simulink model "ThdRwRtStCshnFldIsPosChk"  (R2018b)
settings: Solver=FixedStepDiscrete  StartTime=0.0  StopTime=10.0  FixedStep=0.01  RelTol=1e-3
undefined symbols (not defined in the file or in its folder): KeSMSuThrdRwCushFoldPosDelta_Val, KeSMSuThrdRwCushFoldPosTolr_Val, KeSMSuVehicleModelConfig_Val
libraries: StIsPosChkLib x8, simulink x5
settings Model: Creator=sn2xws  LastModifiedBy=sn55gm
settings Model: ModifiedHistory=|
  | 2024.3.14
  | V2.3.0
  | Bug 813950 童锁Lock，Mode1_Easy Entry Mode 不应调用失败
  | 2024.6.25
  | V3.0.0 557模式流程V1.6
  | 2024.9.6 V3.0.1 新增Md56
  | 2025.2.19 V3.8.0 Bug 991386 Md1 三排占座时未移动且报了成功
  | 25.7.1 v3.13.0 新增Md61 Md62
settings DataIOCC: SaveFormat=StructureWithTime
settings OptimizationCC: DefaultParameterBehavior=Inlined  EnhancedBackFolding=on  PassReuseOutputArgsAs=Individual arguments  ZeroExternalMemoryAtStartup=off  ZeroInternalMemoryAtStartup=off  OptimizeBlockOrder=speed  DifferentSizesBufferReuse=on  OptimizationCustomize=off
settings DebuggingCC: ParameterTunabilityLossMsg=error
settings ModelReferenceCC: ModelReferenceNumInstancesAllowed=Single
settings SFSimCC: MATLABDynamicMemAlloc=off
settings RTWCC: SystemTargetFile=autosar.tlc  GenCodeOnly=on  TemplateMakefile=ert_default_tmf  Description=AUTOSAR  GenerateReport=on  IncludeHyperlinkInReport=on  LaunchReport=on  GenerateTraceInfo=on  GenerateTraceReport=on  GenerateTraceReportSl=on  GenerateTraceReportSf=on  GenerateTraceReportEml=on
settings CodeAppCC: ForceParamTrailComments=on  IgnoreCustomStorageClasses=off  OperatorAnnotations=on  SimulinkDataObjDesc=on  SFDataObjDesc=on  InsertBlockDesc=on
settings STFCustomTargetCC: TargetLangStandard=C99 (ISO)  MultiwordLength=256  ParMdlRefBuildCompliant=on  CompOptLevelCompliant=on  IncludeMdlTerminateFcn=off  CombineOutputUpdateFcns=on  SuppressErrorStatus=on  ERTCustomFileBanners=on  SupportNonFinite=off  SupportComplex=off  SupportContinuousTime=off  SupportNonInlinedSFcns=off  RemoveResetFunc=on  MATLABClassNameForMDSCustomization=Simulink.SoftwareTarget.ERTCustomization  AutosarCompliant=on  UseToolchainInfoCompliant=on  LookupTableObjectStructAxisOrder=2,1,3,4,...  LUTObjectStructOrderEvenSpacing=Size,Table,Breakpoints  SystemTargetFile=autosar.tlc
settings ERTTargetCC: TargetLangStandard=C99 (ISO)  ConcurrentExecutionCompliant=off  IncludeMdlTerminateFcn=off  SuppressErrorStatus=on  SupportNonFinite=off  SupportComplex=off  ModelStepFunctionPrototypeControlCompliant=off  CPPClassGenCompliant=off  AutosarCompliant=on  LookupTableObjectStructAxisOrder=2,1,3,4,...  LUTObjectStructOrderEvenSpacing=Size,Table,Breakpoints  InlinedParameterPlacement=NonHierarchical  ERTCustomFileTemplate=example_file_process.tlc  ERTFilePackagingFormat=Compact

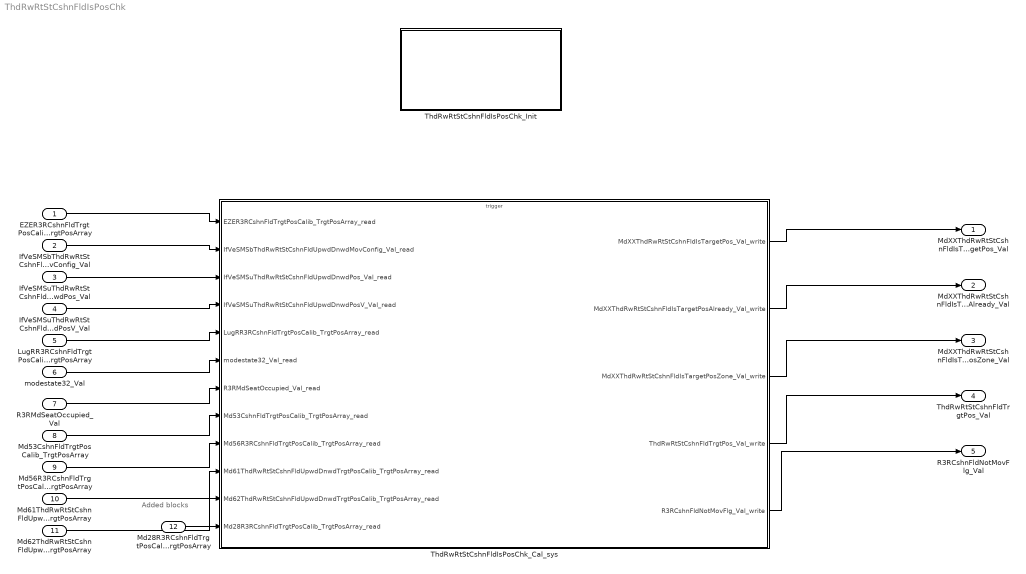
== system ThdRwRtStCshnFldIsPosChk ==
  note: Added blocks
  EZER3RCshnFldTrgtPosCalib_TrgtPosArray : Inport  Description=|  OutDataTypeStr=uint16  PortDimensions=3
      | 0:Pos
      | 1:Max
      | 2:Min
  IfVeSMSbThdRwRtStCshnFldUpwdDnwdMovConfig_Val : Inport  Port=2  OutDataTypeStr=boolean  PortDimensions=1
  IfVeSMSuThdRwRtStCshnFldUpwdDnwdPos_Val : Inport  Port=3  OutDataTypeStr=uint16  PortDimensions=1
  IfVeSMSuThdRwRtStCshnFldUpwdDnwdPosV_Val : Inport  Port=4  OutDataTypeStr=boolean  PortDimensions=1
  LugRR3RCshnFldTrgtPosCalib_TrgtPosArray : Inport  Description=|  Port=5  OutDataTypeStr=uint16  PortDimensions=3
      | 0:Pos
      | 1:Max
      | 2:Min
  modestate32_Val : Inport  Port=6  OutDataTypeStr=uint32  PortDimensions=1
  R3RMdSeatOccupied_Val : Inport  Port=7  OutDataTypeStr=boolean  PortDimensions=1
  Md53CshnFldTrgtPosCalib_TrgtPosArray : Inport  Description=|  Port=8  OutDataTypeStr=uint16  PortDimensions=3
      | 0:Pos
      | 1:Max
      | 2:Min
  Md56R3RCshnFldTrgtPosCalib_TrgtPosArray : Inport  Description=|  Port=9  OutDataTypeStr=uint16  PortDimensions=3
      | 0:Pos
      | 1:Max
      | 2:Min
  Md61ThdRwRtStCshnFldUpwdDnwdTrgtPosCalib_TrgtPosArray : Inport  Description=|  Port=10  OutDataTypeStr=uint16  PortDimensions=3
      | 0:Pos
      | 1:Max
      | 2:Min
  Md62ThdRwRtStCshnFldUpwdDnwdTrgtPosCalib_TrgtPosArray : Inport  Description=|  Port=11  OutDataTypeStr=uint16  PortDimensions=3
      | 0:Pos
      | 1:Max
      | 2:Min
  Md28R3RCshnFldTrgtPosCalib_TrgtPosArray : Inport  Description=|  Port=12  OutDataTypeStr=uint16  PortDimensions=3
      | 0:Pos
      | 1:Max
      | 2:Min
  ThdRwRtStCshnFldIsPosChk_Cal_sys : Subsystem
  ThdRwRtStCshnFldIsPosChk_Init : Subsystem
  MdXXThdRwRtStCshnFldIsTargetPos_Val : Outport  OutDataTypeStr=uint32  PortDimensions=1
  MdXXThdRwRtStCshnFldIsTargetPosAlready_Val : Outport  Port=2  OutDataTypeStr=uint32  PortDimensions=1
  MdXXThdRwRtStCshnFldIsTargetPosZone_Val : Outport  Port=3  OutDataTypeStr=uint32  PortDimensions=1
  ThdRwRtStCshnFldTrgtPos_Val : Outport  Port=4  OutDataTypeStr=uint16  PortDimensions=1
  R3RCshnFldNotMovFlg_Val : Outport  Port=5  OutDataTypeStr=boolean  PortDimensions=1
  wires:
  EZER3RCshnFldTrgtPosCalib_TrgtPosArray/1 -> ThdRwRtStCshnFldIsPosChk_Cal_sys/1(EZER3RCshnFldTrgtPosCalib_TrgtPosArray_read)
  IfVeSMSbThdRwRtStCshnFldUpwdDnwdMovConfig_Val/1 -> ThdRwRtStCshnFldIsPosChk_Cal_sys/2(IfVeSMSbThdRwRtStCshnFldUpwdDnwdMovConfig_Val_read)
  IfVeSMSuThdRwRtStCshnFldUpwdDnwdPos_Val/1 -> ThdRwRtStCshnFldIsPosChk_Cal_sys/3(IfVeSMSuThdRwRtStCshnFldUpwdDnwdPos_Val_read)
  IfVeSMSuThdRwRtStCshnFldUpwdDnwdPosV_Val/1 -> ThdRwRtStCshnFldIsPosChk_Cal_sys/4(IfVeSMSuThdRwRtStCshnFldUpwdDnwdPosV_Val_read)
  LugRR3RCshnFldTrgtPosCalib_TrgtPosArray/1 -> ThdRwRtStCshnFldIsPosChk_Cal_sys/5(LugRR3RCshnFldTrgtPosCalib_TrgtPosArray_read)
  modestate32_Val/1 -> ThdRwRtStCshnFldIsPosChk_Cal_sys/6(modestate32_Val_read)
  ThdRwRtStCshnFldIsPosChk_Cal_sys/1(MdXXThdRwRtStCshnFldIsTargetPos_Val_write) -> MdXXThdRwRtStCshnFldIsTargetPos_Val/1
  ThdRwRtStCshnFldIsPosChk_Cal_sys/2(MdXXThdRwRtStCshnFldIsTargetPosAlready_Val_write) -> MdXXThdRwRtStCshnFldIsTargetPosAlready_Val/1
  ThdRwRtStCshnFldIsPosChk_Cal_sys/3(MdXXThdRwRtStCshnFldIsTargetPosZone_Val_write) -> MdXXThdRwRtStCshnFldIsTargetPosZone_Val/1
  ThdRwRtStCshnFldIsPosChk_Cal_sys/4(ThdRwRtStCshnFldTrgtPos_Val_write) -> ThdRwRtStCshnFldTrgtPos_Val/1
  R3RMdSeatOccupied_Val/1 -> ThdRwRtStCshnFldIsPosChk_Cal_sys/7(R3RMdSeatOccupied_Val_read)
  Md53CshnFldTrgtPosCalib_TrgtPosArray/1 -> ThdRwRtStCshnFldIsPosChk_Cal_sys/8(Md53CshnFldTrgtPosCalib_TrgtPosArray_read)
  ThdRwRtStCshnFldIsPosChk_Cal_sys/5(R3RCshnFldNotMovFlg_Val_write) -> R3RCshnFldNotMovFlg_Val/1
  Md56R3RCshnFldTrgtPosCalib_TrgtPosArray/1 -> ThdRwRtStCshnFldIsPosChk_Cal_sys/9(Md56R3RCshnFldTrgtPosCalib_TrgtPosArray_read)
  Md61ThdRwRtStCshnFldUpwdDnwdTrgtPosCalib_TrgtPosArray/1 -> ThdRwRtStCshnFldIsPosChk_Cal_sys/10(Md61ThdRwRtStCshnFldUpwdDnwdTrgtPosCalib_TrgtPosArray_read)
  Md62ThdRwRtStCshnFldUpwdDnwdTrgtPosCalib_TrgtPosArray/1 -> ThdRwRtStCshnFldIsPosChk_Cal_sys/11(Md62ThdRwRtStCshnFldUpwdDnwdTrgtPosCalib_TrgtPosArray_read)
  Md28R3RCshnFldTrgtPosCalib_TrgtPosArray/1 -> ThdRwRtStCshnFldIsPosChk_Cal_sys/12(Md28R3RCshnFldTrgtPosCalib_TrgtPosArray_read)

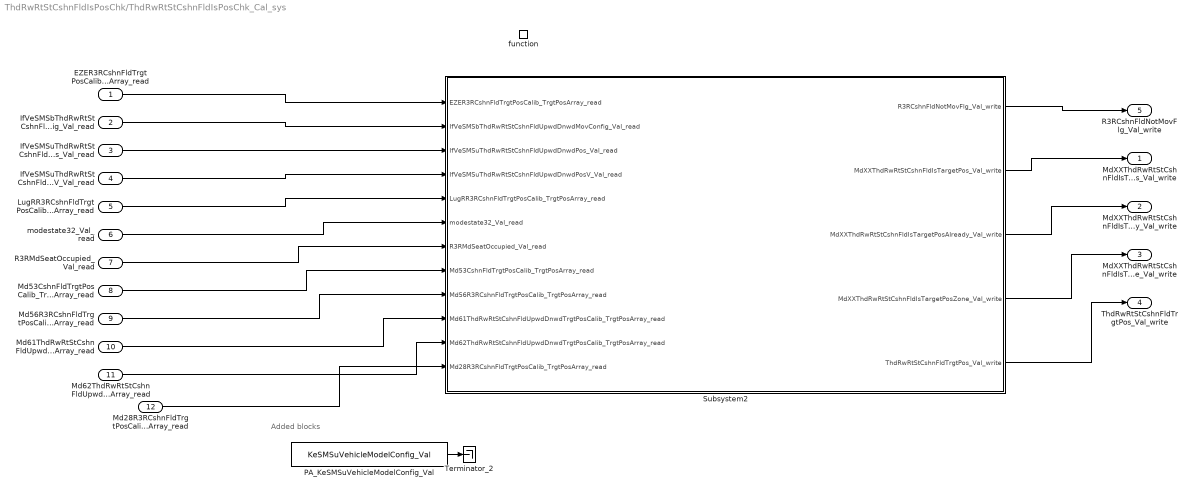
== system ThdRwRtStCshnFldIsPosChk/ThdRwRtStCshnFldIsPosChk_Cal_sys ==
  note: Added blocks
  EZER3RCshnFldTrgtPosCalib_TrgtPosArray_read : Inport
  IfVeSMSbThdRwRtStCshnFldUpwdDnwdMovConfig_Val_read : Inport  Port=2
  IfVeSMSuThdRwRtStCshnFldUpwdDnwdPos_Val_read : Inport  Port=3
  IfVeSMSuThdRwRtStCshnFldUpwdDnwdPosV_Val_read : Inport  Port=4
  LugRR3RCshnFldTrgtPosCalib_TrgtPosArray_read : Inport  Port=5
  modestate32_Val_read : Inport  Port=6
  R3RMdSeatOccupied_Val_read : Inport  Port=7
  Md53CshnFldTrgtPosCalib_TrgtPosArray_read : Inport  Port=8
  Md56R3RCshnFldTrgtPosCalib_TrgtPosArray_read : Inport  Port=9
  Md61ThdRwRtStCshnFldUpwdDnwdTrgtPosCalib_TrgtPosArray_read : Inport  Port=10
  Md62ThdRwRtStCshnFldUpwdDnwdTrgtPosCalib_TrgtPosArray_read : Inport  Port=11
  Md28R3RCshnFldTrgtPosCalib_TrgtPosArray_read : Inport  Port=12
  function : TriggerPort  TriggerType=function-call  IsSimulinkFunction=on  FunctionName=ThdRwRtStCshnFldIsPosChk_Cal  VariantControl=(inherit)
  PA_KeSMSuVehicleModelConfig_Val : Constant  Value=KeSMSuVehicleModelConfig_Val
  Subsystem2 : Subsystem
  Terminator_2 : Terminator
  MdXXThdRwRtStCshnFldIsTargetPos_Val_write : Outport
      settings: EnsureOutportIsVirtual=on
  MdXXThdRwRtStCshnFldIsTargetPosAlready_Val_write : Outport  Port=2
      settings: EnsureOutportIsVirtual=on
  MdXXThdRwRtStCshnFldIsTargetPosZone_Val_write : Outport  Port=3
      settings: EnsureOutportIsVirtual=on
  ThdRwRtStCshnFldTrgtPos_Val_write : Outport  Port=4
      settings: EnsureOutportIsVirtual=on
  R3RCshnFldNotMovFlg_Val_write : Outport  Port=5
      settings: EnsureOutportIsVirtual=on
  wires:
  Subsystem2/5(ThdRwRtStCshnFldTrgtPos_Val_write) -> ThdRwRtStCshnFldTrgtPos_Val_write/1
  Subsystem2/2(MdXXThdRwRtStCshnFldIsTargetPos_Val_write) -> MdXXThdRwRtStCshnFldIsTargetPos_Val_write/1
  Subsystem2/3(MdXXThdRwRtStCshnFldIsTargetPosAlready_Val_write) -> MdXXThdRwRtStCshnFldIsTargetPosAlready_Val_write/1
  Subsystem2/4(MdXXThdRwRtStCshnFldIsTargetPosZone_Val_write) -> MdXXThdRwRtStCshnFldIsTargetPosZone_Val_write/1
  EZER3RCshnFldTrgtPosCalib_TrgtPosArray_read/1 -> Subsystem2/1(EZER3RCshnFldTrgtPosCalib_TrgtPosArray_read)
  IfVeSMSbThdRwRtStCshnFldUpwdDnwdMovConfig_Val_read/1 -> Subsystem2/2(IfVeSMSbThdRwRtStCshnFldUpwdDnwdMovConfig_Val_read)
  IfVeSMSuThdRwRtStCshnFldUpwdDnwdPos_Val_read/1 -> Subsystem2/3(IfVeSMSuThdRwRtStCshnFldUpwdDnwdPos_Val_read)
  IfVeSMSuThdRwRtStCshnFldUpwdDnwdPosV_Val_read/1 -> Subsystem2/4(IfVeSMSuThdRwRtStCshnFldUpwdDnwdPosV_Val_read)
  LugRR3RCshnFldTrgtPosCalib_TrgtPosArray_read/1 -> Subsystem2/5(LugRR3RCshnFldTrgtPosCalib_TrgtPosArray_read)
  modestate32_Val_read/1 -> Subsystem2/6(modestate32_Val_read)
  R3RMdSeatOccupied_Val_read/1 -> Subsystem2/7(R3RMdSeatOccupied_Val_read)
  Md53CshnFldTrgtPosCalib_TrgtPosArray_read/1 -> Subsystem2/8(Md53CshnFldTrgtPosCalib_TrgtPosArray_read)
  Subsystem2/1(R3RCshnFldNotMovFlg_Val_write) -> R3RCshnFldNotMovFlg_Val_write/1
  Md56R3RCshnFldTrgtPosCalib_TrgtPosArray_read/1 -> Subsystem2/9(Md56R3RCshnFldTrgtPosCalib_TrgtPosArray_read)
  Md61ThdRwRtStCshnFldUpwdDnwdTrgtPosCalib_TrgtPosArray_read/1 -> Subsystem2/10(Md61ThdRwRtStCshnFldUpwdDnwdTrgtPosCalib_TrgtPosArray_read)
  Md62ThdRwRtStCshnFldUpwdDnwdTrgtPosCalib_TrgtPosArray_read/1 -> Subsystem2/11(Md62ThdRwRtStCshnFldUpwdDnwdTrgtPosCalib_TrgtPosArray_read)
  Md28R3RCshnFldTrgtPosCalib_TrgtPosArray_read/1 -> Subsystem2/12(Md28R3RCshnFldTrgtPosCalib_TrgtPosArray_read)
  PA_KeSMSuVehicleModelConfig_Val/1 -> Terminator_2/1

== system ThdRwRtStCshnFldIsPosChk/ThdRwRtStCshnFldIsPosChk_Init ==
  note: Added blocks
  note: Added blocks
  note: Added blocks
  Event Listener : EventListener  EventName=reset
  PA_KeSMSuThrdRwCushFoldPosDelta_Val : Constant  Value=KeSMSuThrdRwCushFoldPosDelta_Val
  PA_KeSMSuThrdRwCushFoldPosTolr_Val : Constant  Value=KeSMSuThrdRwCushFoldPosTolr_Val
  PA_KeSMSuVehicleModelConfig_Val : Constant  Value=KeSMSuVehicleModelConfig_Val
  Terminator_1 : Terminator
  Terminator_2 : Terminator
  Terminator_3 : Terminator
  wires:
  PA_KeSMSuThrdRwCushFoldPosDelta_Val/1 -> Terminator_1/1
  PA_KeSMSuThrdRwCushFoldPosTolr_Val/1 -> Terminator_2/1
  PA_KeSMSuVehicleModelConfig_Val/1 -> Terminator_3/1

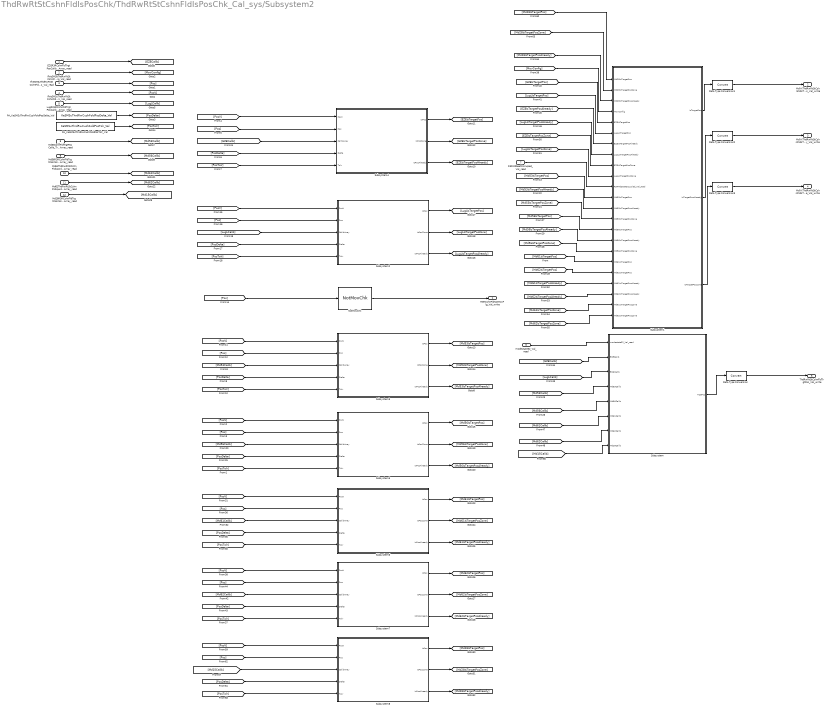
== system ThdRwRtStCshnFldIsPosChk/ThdRwRtStCshnFldIsPosChk_Cal_sys/Subsystem2 ==
  EZER3RCshnFldTrgtPosCalib_TrgtPosArray_read : Inport
  IfVeSMSbThdRwRtStCshnFldUpwdDnwdMovConfig_Val_read : Inport  Port=2
  IfVeSMSuThdRwRtStCshnFldUpwdDnwdPos_Val_read : Inport  Port=3
  IfVeSMSuThdRwRtStCshnFldUpwdDnwdPosV_Val_read : Inport  Port=4
  LugRR3RCshnFldTrgtPosCalib_TrgtPosArray_read : Inport  Port=5
  modestate32_Val_read : Inport  Port=6
  R3RMdSeatOccupied_Val_read : Inport  Port=7
  Md53CshnFldTrgtPosCalib_TrgtPosArray_read : Inport  Port=8
  Md56R3RCshnFldTrgtPosCalib_TrgtPosArray_read : Inport  Port=9
  Md61ThdRwRtStCshnFldUpwdDnwdTrgtPosCalib_TrgtPosArray_read : Inport  Port=10
  Md62ThdRwRtStCshnFldUpwdDnwdTrgtPosCalib_TrgtPosArray_read : Inport  Port=11
  Md28R3RCshnFldTrgtPosCalib_TrgtPosArray_read : Inport  Port=12
  Data Type Conversion{,1..3} (4 alike) : DataTypeConversion
  NotMovChk : StIsPosChkLib/NotMovChk  SystemSampleTime=-1
  PA_KeSMSuThrdRwCushFoldPosDelta_Val : Constant  Value=KeSMSuThrdRwCushFoldPosDelta_Val
  PA_KeSMSuThrdRwCushFoldPosTolr_Val : Constant  Value=KeSMSuThrdRwCushFoldPosTolr_Val
  Subsystem : Subsystem
  Subsystem1 : Subsystem
  Subsystem2 : Subsystem
  Subsystem3 : Subsystem
  Subsystem4 : Subsystem
  Subsystem5 : Subsystem
  Subsystem6 : Subsystem
  Subsystem7 : Subsystem
  Subsystem8 : Subsystem
  R3RCshnFldNotMovFlg_Val_write : Outport
      settings: EnsureOutportIsVirtual=on
  MdXXThdRwRtStCshnFldIsTargetPos_Val_write : Outport  Port=2
      settings: EnsureOutportIsVirtual=on
  MdXXThdRwRtStCshnFldIsTargetPosAlready_Val_write : Outport  Port=3
      settings: EnsureOutportIsVirtual=on
  MdXXThdRwRtStCshnFldIsTargetPosZone_Val_write : Outport  Port=4
      settings: EnsureOutportIsVirtual=on
  ThdRwRtStCshnFldTrgtPos_Val_write : Outport  Port=5
      settings: EnsureOutportIsVirtual=on
  wires:
  [LugLCalib] -> Subsystem/3(EZQCalib)
  Subsystem1/3(IsTargetPosZone) -> Data Type Conversion3/1
  [EZEIsTargetPosZone] -> Subsystem1/9(EZEIsTargetPosZone)
  [EZECalib] -> Subsystem/2(EZECalib)
  NotMovChk/1 -> R3RCshnFldNotMovFlg_Val_write/1
  [EZEIsTargetPosAlready] -> Subsystem1/7(EZEIsTargetPosAlready)
  [LugLIsTargetPosAlready] -> Subsystem1/8(LugLIsTargetPosAlready)
  Subsystem2/2(IsPosZone) -> [LugLIsTargetPosZone]
  modestate32_Val_read/1 -> Subsystem/1(modestate32_Val_read)
  Data Type Conversion1/1 -> MdXXThdRwRtStCshnFldIsTargetPos_Val_write/1
  Subsystem2/1(IsPos) -> [LugLIsTargetPos]
  Subsystem/1(TrgtPos) -> Data Type Conversion/1
  Subsystem4/3(IsPosAlready) -> [EZEIsTargetPosAlready]
  [EZECalib] -> Subsystem4/3(CalibArray)
  [LugLIsTargetPos] -> Subsystem1/6(LugLIsTargetPos)
  [EZEIsTargetPos] -> Subsystem1/5(EZEIsTargetPos)
  Subsystem1/1(IsTargetPos) -> Data Type Conversion1/1
  Subsystem4/1(IsPos) -> [EZEIsTargetPos]
  Data Type Conversion2/1 -> MdXXThdRwRtStCshnFldIsTargetPosAlready_Val_write/1
  [PosV] -> Subsystem4/1(PosV)
  [LugLCalib] -> Subsystem2/3(CalibArray)
  [LugLIsTargetPosZone] -> Subsystem1/10(LugLIsTargetPosZone)
  [PosDelta] -> Subsystem4/4(Delta)
  Data Type Conversion/1 -> ThdRwRtStCshnFldTrgtPos_Val_write/1
  PA_KeSMSuThrdRwCushFoldPosDelta_Val/1 -> [PosDelta]
  [PosDelta] -> Subsystem2/4(Delta)
  EZER3RCshnFldTrgtPosCalib_TrgtPosArray_read/1 -> [EZECalib]
  IfVeSMSbThdRwRtStCshnFldUpwdDnwdMovConfig_Val_read/1 -> [MovConfig]
  IfVeSMSuThdRwRtStCshnFldUpwdDnwdPosV_Val_read/1 -> [PosV]
  IfVeSMSuThdRwRtStCshnFldUpwdDnwdPos_Val_read/1 -> [Pos]
  [PosTolr] -> Subsystem4/5(Tolr)
  Subsystem2/3(IsPosAlready) -> [LugLIsTargetPosAlready]
  LugRR3RCshnFldTrgtPosCalib_TrgtPosArray_read/1 -> [LugLCalib]
  [Pos] -> Subsystem2/2(Pos)
  PA_KeSMSuThrdRwCushFoldPosTolr_Val/1 -> [PosTolr]
  Subsystem4/2(IsPosZone) -> [EZEIsTargetPosZone]
  [PosV] -> Subsystem2/1(PosV)
  Subsystem1/2(IsTargetPosAlready) -> Data Type Conversion2/1
  [PosTolr] -> Subsystem2/5(Tolr)
  [MovConfig] -> Subsystem1/4(MovConfig)
  [Pos] -> NotMovChk/1
  [Pos] -> Subsystem4/2(Pos)
  Data Type Conversion3/1 -> MdXXThdRwRtStCshnFldIsTargetPosZone_Val_write/1
  R3RMdSeatOccupied_Val_read/1 -> Subsystem1/11(R3RMdSeatOccupied_Val_read)
  Md53CshnFldTrgtPosCalib_TrgtPosArray_read/1 -> [Md53Calib]
  [Md53Calib] -> Subsystem3/3(CalibArray)
  [PosTolr] -> Subsystem3/5(Tolr)
  [PosDelta] -> Subsystem3/4(Delta)
  [PosV] -> Subsystem3/1(PosV)
  [Pos] -> Subsystem3/2(Pos)
  Subsystem3/3(IsPosAlready) -> [Md53IsTargetPosAlready]
  Subsystem3/1(IsPos) -> [Md53IsTargetPos]
  Subsystem3/2(IsPosZone) -> [Md53IsTargetPosZone]
  [Md53Calib] -> Subsystem/4(Md53Calib)
  [Md53IsTargetPos] -> Subsystem1/12(Md53IsTargetPos)
  [Md53IsTargetPosAlready] -> Subsystem1/13(Md53IsTargetPosAlready)
  [Md53IsTargetPosZone] -> Subsystem1/14(Md53IsTargetPosZone)
  Md56R3RCshnFldTrgtPosCalib_TrgtPosArray_read/1 -> [Md56Calib]
  Subsystem5/2(IsPosZone) -> [Md56IsTargetPosZone]
  Subsystem5/1(IsPos) -> [Md56IsTargetPos]
  Subsystem5/3(IsPosAlready) -> [Md56IsTargetPosAlready]
  [Pos] -> Subsystem5/2(Pos)
  [PosV] -> Subsystem5/1(PosV)
  [PosDelta] -> Subsystem5/4(Delta)
  [PosTolr] -> Subsystem5/5(Tolr)
  [Md56Calib] -> Subsystem5/3(CalibArray)
  [Md56Calib] -> Subsystem/5(Md56Calib)
  [Md56IsTargetPos] -> Subsystem1/15(Md56IsTargetPos)
  [Md56IsTargetPosAlready] -> Subsystem1/16(Md56IsTargetPosAlready)
  [Md56IsTargetPosZone] -> Subsystem1/17(Md56IsTargetPosZone)
  Md62ThdRwRtStCshnFldUpwdDnwdTrgtPosCalib_TrgtPosArray_read/1 -> [Md62Calib]
  Md61ThdRwRtStCshnFldUpwdDnwdTrgtPosCalib_TrgtPosArray_read/1 -> [Md61Calib]
  [Md61Calib] -> Subsystem6/3(CalibArray)
  [PosTolr] -> Subsystem6/5(Tolr)
  [PosDelta] -> Subsystem6/4(Delta)
  [PosV] -> Subsystem6/1(PosV)
  [Pos] -> Subsystem6/2(Pos)
  Subsystem6/3(IsPosAlready) -> [Md61IsTargetPosAlready]
  Subsystem6/1(IsPos) -> [Md61IsTargetPos]
  Subsystem6/2(IsPosZone) -> [Md61IsTargetPosZone]
  Subsystem7/2(IsPosZone) -> [Md62IsTargetPosZone]
  Subsystem7/1(IsPos) -> [Md62IsTargetPos]
  Subsystem7/3(IsPosAlready) -> [Md62IsTargetPosAlready]
  [Pos] -> Subsystem7/2(Pos)
  [PosV] -> Subsystem7/1(PosV)
  [PosDelta] -> Subsystem7/4(Delta)
  [PosTolr] -> Subsystem7/5(Tolr)
  [Md62Calib] -> Subsystem7/3(CalibArray)
  [Md62Calib] -> Subsystem/7(Md62Calib)
  [Md61Calib] -> Subsystem/6(Md61Calib)
  [Md61IsTargetPos] -> Subsystem1/18(Md61IsTargetPos)
  [Md62IsTargetPos] -> Subsystem1/19(Md62IsTargetPos)
  [Md61IsTargetPosAlready] -> Subsystem1/20(Md61IsTargetPosAlready)
  [Md62IsTargetPosAlready] -> Subsystem1/21(Md62IsTargetPosAlready)
  [Md61IsTargetPosZone] -> Subsystem1/22(Md61IsTargetPosZone)
  [Md62IsTargetPosZone] -> Subsystem1/23(Md62IsTargetPosZone)
  Md28R3RCshnFldTrgtPosCalib_TrgtPosArray_read/1 -> [Md15Calib]
  [PosTolr] -> Subsystem8/5(Tolr)
  Subsystem8/3(IsPosAlready) -> [Md28IsTargetPosAlready]
  [PosV] -> Subsystem8/1(PosV)
  [Pos] -> Subsystem8/2(Pos)
  [PosDelta] -> Subsystem8/4(Delta)
  [Md15Calib] -> Subsystem8/3(CalibArray)
  Subsystem8/1(IsPos) -> [Md28IsTargetPos]
  Subsystem8/2(IsPosZone) -> [Md28IsTargetPosZone]
  [Md28IsTargetPosAlready] -> Subsystem1/3(Md28IsTargetPosAlready)
  [Md28IsTargetPosZone] -> Subsystem1/2(Md28IsTargetPosZone)
  [Md28IsTargetPos] -> Subsystem1/1(Md28IsTargetPos)
  [Md15Calib] -> Subsystem/8(Md28Calib)

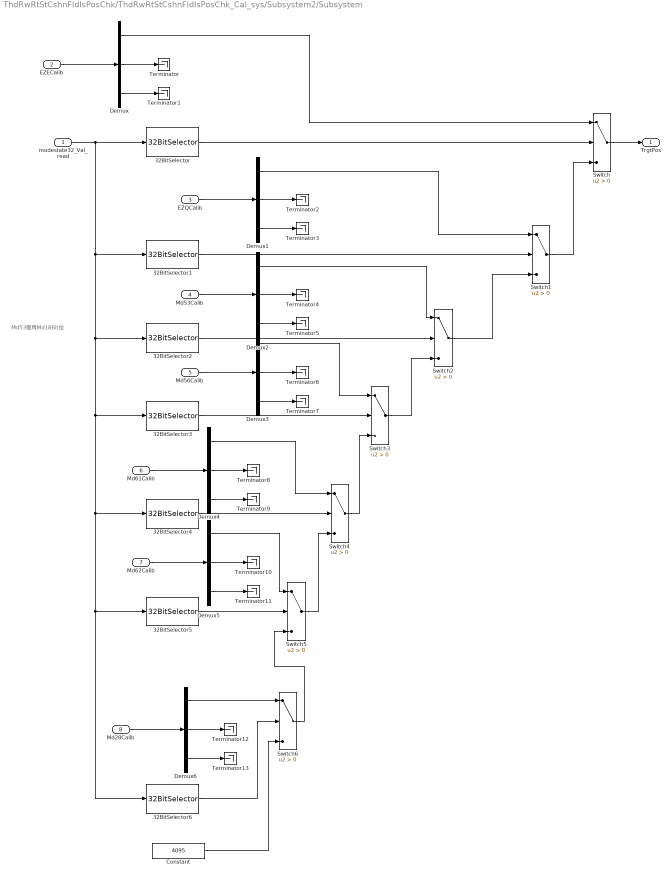
== system ThdRwRtStCshnFldIsPosChk/ThdRwRtStCshnFldIsPosChk_Cal_sys/Subsystem2/Subsystem ==
  note: Md53借用Md18Bit位
  modestate32_Val_read : Inport
  EZECalib : Inport  Port=2
  EZQCalib : Inport  Port=3
  Md53Calib : Inport  Port=4
  Md56Calib : Inport  Port=5
  Md61Calib : Inport  Port=6
  Md62Calib : Inport  Port=7
  Md28Calib : Inport  Port=8
  32BitSelector : StIsPosChkLib/32BitSelector  BitNum=0
  32BitSelector1 : StIsPosChkLib/32BitSelector  BitNum=8
  32BitSelector2 : StIsPosChkLib/32BitSelector  BitNum=17
  32BitSelector3 : StIsPosChkLib/32BitSelector  BitNum=24
  32BitSelector4 : StIsPosChkLib/32BitSelector  BitNum=5
  32BitSelector5 : StIsPosChkLib/32BitSelector  BitNum=6
  32BitSelector6 : StIsPosChkLib/32BitSelector  BitNum=14
  Constant : Constant  Value=4095  OutDataTypeStr=uint16
  Demux{,1..6} (7 alike) : Demux  Outputs=3
  Switch{,1..6} (7 alike) : Switch  Criteria=u2 > Threshold
  Terminator{,1..13} (14 alike) : Terminator
  TrgtPos : Outport
      settings: EnsureOutportIsVirtual=on
  wires:
  32BitSelector/1 -> Switch/2
  modestate32_Val_read/1 -> 32BitSelector2/1, 32BitSelector6/1, 32BitSelector5/1, 32BitSelector4/1, 32BitSelector3/1, 32BitSelector1/1, 32BitSelector/1
  Demux/1 -> Switch/1
  Demux/3 -> Terminator1/1
  Demux/2 -> Terminator/1
  EZECalib/1 -> Demux/1
  EZQCalib/1 -> Demux1/1
  Demux1/2 -> Terminator2/1
  Demux1/3 -> Terminator3/1
  Demux1/1 -> Switch1/1
  Switch/1 -> TrgtPos/1
  Switch1/1 -> Switch/3
  Switch2/1 -> Switch1/3
  32BitSelector1/1 -> Switch1/2
  32BitSelector2/1 -> Switch2/2
  Demux2/1 -> Switch2/1
  Demux2/3 -> Terminator5/1
  Demux2/2 -> Terminator4/1
  Md53Calib/1 -> Demux2/1
  Switch3/1 -> Switch2/3
  32BitSelector3/1 -> Switch3/2
  Md56Calib/1 -> Demux3/1
  Demux3/2 -> Terminator6/1
  Demux3/3 -> Terminator7/1
  Demux3/1 -> Switch3/1
  Switch4/1 -> Switch3/3
  Switch5/1 -> Switch4/3
  32BitSelector4/1 -> Switch4/2
  32BitSelector5/1 -> Switch5/2
  Demux4/3 -> Terminator9/1
  Demux4/2 -> Terminator8/1
  Md61Calib/1 -> Demux4/1
  Demux4/1 -> Switch4/1
  Md62Calib/1 -> Demux5/1
  Demux5/2 -> Terminator10/1
  Demux5/1 -> Switch5/1
  Demux5/3 -> Terminator11/1
  Demux6/3 -> Terminator13/1
  Demux6/2 -> Terminator12/1
  Demux6/1 -> Switch6/1
  Md28Calib/1 -> Demux6/1
  32BitSelector6/1 -> Switch6/2
  Constant/1 -> Switch6/3
  Switch6/1 -> Switch5/3

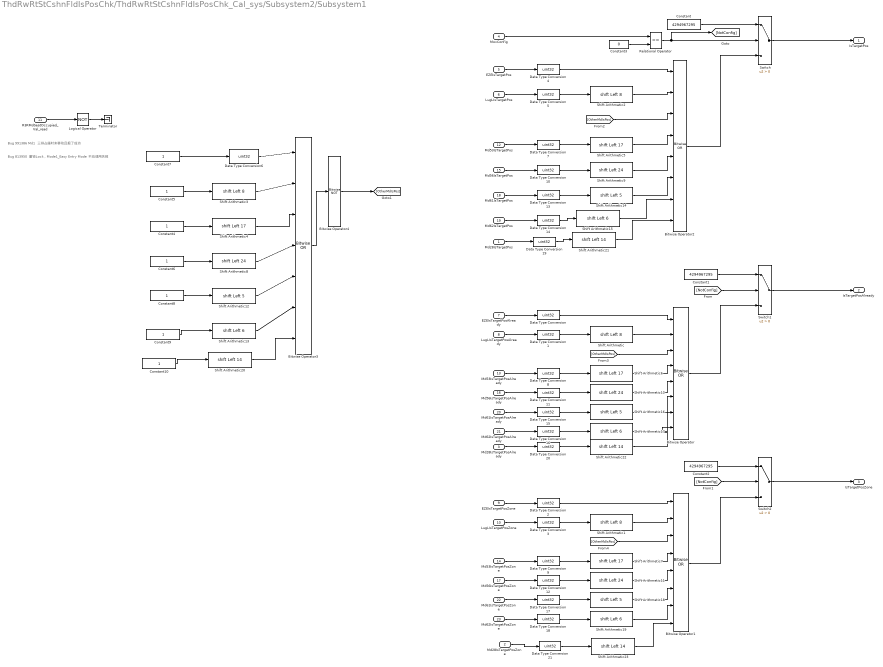
== system ThdRwRtStCshnFldIsPosChk/ThdRwRtStCshnFldIsPosChk_Cal_sys/Subsystem2/Subsystem1 ==
  note: Bug 991386 Md1 三排占座时未移动且报了成功
  note: Bug 813950 童锁Lock，Mode1_Easy Entry Mode 不应调用失败
  Md28IsTargetPos : Inport
  Md28IsTargetPosZone : Inport  Port=2
  Md28IsTargetPosAlready : Inport  Port=3
  MovConfig : Inport  Port=4
  EZEIsTargetPos : Inport  Port=5
  LugLIsTargetPos : Inport  Port=6
  EZEIsTargetPosAlready : Inport  Port=7
  LugLIsTargetPosAlready : Inport  Port=8
  EZEIsTargetPosZone : Inport  Port=9
  LugLIsTargetPosZone : Inport  Port=10
  R3RMdSeatOccupied_Val_read : Inport  Port=11
  Md53IsTargetPos : Inport  Port=12
  Md53IsTargetPosAlready : Inport  Port=13
  Md53IsTargetPosZone : Inport  Port=14
  Md56IsTargetPos : Inport  Port=15
  Md56IsTargetPosAlready : Inport  Port=16
  Md56IsTargetPosZone : Inport  Port=17
  Md61IsTargetPos : Inport  Port=18
  Md62IsTargetPos : Inport  Port=19
  Md61IsTargetPosAlready : Inport  Port=20
  Md62IsTargetPosAlready : Inport  Port=21
  Md61IsTargetPosZone : Inport  Port=22
  Md62IsTargetPosZone : Inport  Port=23
  Bitwise Operator : simulink/Logic and Bit Operations/Bitwise Operator  logicop=OR  UseBitMask=off  NumInputPorts=8  BitMask=bin2dec('11011001')  BitMaskRealWorld=Stored Integer
  Bitwise Operator1 : simulink/Logic and Bit Operations/Bitwise Operator  logicop=OR  UseBitMask=off  NumInputPorts=8  BitMask=bin2dec('11011001')  BitMaskRealWorld=Stored Integer
  Bitwise Operator2 : simulink/Logic and Bit Operations/Bitwise Operator  logicop=OR  UseBitMask=off  NumInputPorts=8  BitMask=bin2dec('11011001')  BitMaskRealWorld=Stored Integer
  Bitwise Operator3 : simulink/Logic and Bit Operations/Bitwise Operator  logicop=OR  UseBitMask=off  NumInputPorts=7  BitMask=bin2dec('11011001')  BitMaskRealWorld=Stored Integer
  Bitwise Operator4 : simulink/Logic and Bit Operations/Bitwise Operator  logicop=NOT  UseBitMask=off  BitMask=bin2dec('11011001')  BitMaskRealWorld=Stored Integer
  Constant : Constant  Value=4294967295  OutDataTypeStr=uint32
  Constant1 : Constant  Value=4294967295  OutDataTypeStr=uint32
  Constant{4..10} (7 alike) : Constant  OutDataTypeStr=uint32
  Constant2 : Constant  Value=4294967295  OutDataTypeStr=uint32
  Constant3 : Constant  Value=0  OutDataTypeStr=uint8
  Data Type Conversion{,1..21} (22 alike) : DataTypeConversion  OutDataTypeStr=uint32
  Logical Operator : Logic  Operator=NOT  AllPortsSameDT=off  OutDataTypeStr=boolean
  Relational Operator : RelationalOperator  Operator===  OutDataTypeStr=boolean  RndMeth=Simplest
  Shift Arithmetic{,1..3} (4 alike) : ArithShift  BitShiftNumber=8  BitShiftDirection=Left
  Shift Arithmetic{8..11} (4 alike) : ArithShift  BitShiftNumber=24  BitShiftDirection=Left
  Shift Arithmetic{12,14,16,18} (4 alike) : ArithShift  BitShiftNumber=5  BitShiftDirection=Left
  Shift Arithmetic{13,15,17,19} (4 alike) : ArithShift  BitShiftNumber=6  BitShiftDirection=Left
  Shift Arithmetic{20..23} (4 alike) : ArithShift  BitShiftNumber=14  BitShiftDirection=Left
  Shift Arithmetic{4..7} (4 alike) : ArithShift  BitShiftNumber=17  BitShiftDirection=Left
  Switch : Switch  Criteria=u2 > Threshold
  Switch1 : Switch  Criteria=u2 > Threshold
  Switch2 : Switch  Criteria=u2 > Threshold
  Terminator : Terminator
  IsTargetPos : Outport
      settings: EnsureOutportIsVirtual=on
  IsTargetPosAlready : Outport  Port=2
      settings: EnsureOutportIsVirtual=on
  IsTargetPosZone : Outport  Port=3
      settings: EnsureOutportIsVirtual=on
  wires:
  Constant3/1 -> Relational Operator/2
  Constant/1 -> Switch/1
  Relational Operator/1 -> [NotConfig], Switch/2
  MovConfig/1 -> Relational Operator/1
  Switch/1 -> IsTargetPos/1
  [NotConfig] -> Switch1/2
  Constant1/1 -> Switch1/1
  Switch1/1 -> IsTargetPosAlready/1
  Switch2/1 -> IsTargetPosZone/1
  Constant2/1 -> Switch2/1
  [NotConfig] -> Switch2/2
  Data Type Conversion1/1 -> Shift Arithmetic/1
  Data Type Conversion/1 -> Bitwise Operator/1
  Shift Arithmetic/1 -> Bitwise Operator/2
  Shift Arithmetic1/1 -> Bitwise Operator1/2
  Data Type Conversion2/1 -> Bitwise Operator1/1
  Data Type Conversion3/1 -> Shift Arithmetic1/1
  Bitwise Operator1/1 -> Switch2/3
  Bitwise Operator/1 -> Switch1/3
  Shift Arithmetic2/1 -> Bitwise Operator2/2
  Data Type Conversion4/1 -> Bitwise Operator2/1
  Data Type Conversion5/1 -> Shift Arithmetic2/1
  Bitwise Operator2/1 -> Switch/3
  EZEIsTargetPos/1 -> Data Type Conversion4/1
  LugLIsTargetPos/1 -> Data Type Conversion5/1
  LugLIsTargetPosZone/1 -> Data Type Conversion3/1
  EZEIsTargetPosZone/1 -> Data Type Conversion2/1
  LugLIsTargetPosAlready/1 -> Data Type Conversion1/1
  EZEIsTargetPosAlready/1 -> Data Type Conversion/1
  Constant5/1 -> Shift Arithmetic3/1
  Shift Arithmetic3/1 -> Bitwise Operator3/2
  Bitwise Operator3/1 -> Bitwise Operator4/1
  Bitwise Operator4/1 -> [OtherMdIsPos]
  [OtherMdIsPos] -> Bitwise Operator2/3
  [OtherMdIsPos] -> Bitwise Operator/3
  [OtherMdIsPos] -> Bitwise Operator1/3
  Data Type Conversion6/1 -> Bitwise Operator3/1
  R3RMdSeatOccupied_Val_read/1 -> Logical Operator/1
  Constant4/1 -> Shift Arithmetic4/1
  Shift Arithmetic4/1 -> Bitwise Operator3/3
  Md53IsTargetPos/1 -> Data Type Conversion7/1
  Data Type Conversion7/1 -> Shift Arithmetic5/1
  Shift Arithmetic5/1 -> Bitwise Operator2/4
  Md53IsTargetPosAlready/1 -> Data Type Conversion8/1
  Data Type Conversion8/1 -> Shift Arithmetic6/1
  Shift Arithmetic6/1 -> Bitwise Operator/4
  Md53IsTargetPosZone/1 -> Data Type Conversion9/1
  Data Type Conversion9/1 -> Shift Arithmetic7/1
  Shift Arithmetic7/1 -> Bitwise Operator1/4
  Shift Arithmetic8/1 -> Bitwise Operator3/4
  Constant6/1 -> Shift Arithmetic8/1
  Shift Arithmetic9/1 -> Bitwise Operator2/5
  Data Type Conversion10/1 -> Shift Arithmetic9/1
  Md56IsTargetPos/1 -> Data Type Conversion10/1
  Shift Arithmetic10/1 -> Bitwise Operator/5
  Data Type Conversion11/1 -> Shift Arithmetic10/1
  Md56IsTargetPosAlready/1 -> Data Type Conversion11/1
  Shift Arithmetic11/1 -> Bitwise Operator1/5
  Data Type Conversion12/1 -> Shift Arithmetic11/1
  Md56IsTargetPosZone/1 -> Data Type Conversion12/1
  Logical Operator/1 -> Terminator/1
  Constant7/1 -> Data Type Conversion6/1
  Constant8/1 -> Shift Arithmetic12/1
  Shift Arithmetic12/1 -> Bitwise Operator3/5
  Shift Arithmetic13/1 -> Bitwise Operator3/6
  Constant9/1 -> Shift Arithmetic13/1
  Md61IsTargetPos/1 -> Data Type Conversion13/1
  Data Type Conversion13/1 -> Shift Arithmetic14/1
  Shift Arithmetic14/1 -> Bitwise Operator2/6
  Shift Arithmetic15/1 -> Bitwise Operator2/7
  Data Type Conversion14/1 -> Shift Arithmetic15/1
  Md62IsTargetPos/1 -> Data Type Conversion14/1
  Md61IsTargetPosAlready/1 -> Data Type Conversion15/1
  Data Type Conversion15/1 -> Shift Arithmetic16/1
  Shift Arithmetic16/1 -> Bitwise Operator/6
  Shift Arithmetic17/1 -> Bitwise Operator/7
  Data Type Conversion16/1 -> Shift Arithmetic17/1
  Md62IsTargetPosAlready/1 -> Data Type Conversion16/1
  Md61IsTargetPosZone/1 -> Data Type Conversion17/1
  Data Type Conversion17/1 -> Shift Arithmetic18/1
  Shift Arithmetic18/1 -> Bitwise Operator1/6
  Shift Arithmetic19/1 -> Bitwise Operator1/7
  Data Type Conversion18/1 -> Shift Arithmetic19/1
  Md62IsTargetPosZone/1 -> Data Type Conversion18/1
  Constant10/1 -> Shift Arithmetic20/1
  Shift Arithmetic20/1 -> Bitwise Operator3/7
  Shift Arithmetic21/1 -> Bitwise Operator2/8
  Data Type Conversion19/1 -> Shift Arithmetic21/1
  Md28IsTargetPos/1 -> Data Type Conversion19/1
  Shift Arithmetic22/1 -> Bitwise Operator/8
  Data Type Conversion20/1 -> Shift Arithmetic22/1
  Md28IsTargetPosAlready/1 -> Data Type Conversion20/1
  Data Type Conversion21/1 -> Shift Arithmetic23/1
  Md28IsTargetPosZone/1 -> Data Type Conversion21/1
  Shift Arithmetic23/1 -> Bitwise Operator1/8

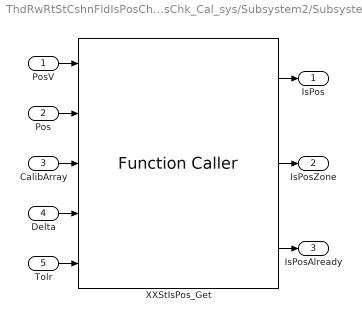
== system ThdRwRtStCshnFldIsPosChk/ThdRwRtStCshnFldIsPosChk_Cal_sys/Subsystem2/Subsystem2 ==
  PosV : Inport
  Pos : Inport  Port=2
  CalibArray : Inport  Port=3
  Delta : Inport  Port=4
  Tolr : Inport  Port=5
  XXStIsPos_Get : FunctionCaller  FunctionPrototype=[IsPos,IsPosZone,IsPosAlready] = XXStIsPos_Get(PosV,Pos,CalibArray,Delta,Tolr)  InputArgumentSpecifications=boolean(true), uint16(1), uint16([1;1;1]), uint16(1), uint16(1)  OutputArgumentSpecifications=boolean(true), boolean(true), boolean(true)
  IsPos : Outport
  IsPosZone : Outport  Port=2
  IsPosAlready : Outport  Port=3
  wires:
  PosV/1 -> XXStIsPos_Get/1
  XXStIsPos_Get/3 -> IsPosAlready/1
  Tolr/1 -> XXStIsPos_Get/5
  XXStIsPos_Get/1 -> IsPos/1
  XXStIsPos_Get/2 -> IsPosZone/1
  CalibArray/1 -> XXStIsPos_Get/3
  Delta/1 -> XXStIsPos_Get/4
  Pos/1 -> XXStIsPos_Get/2

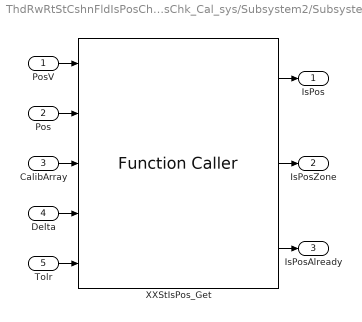
== system ThdRwRtStCshnFldIsPosChk/ThdRwRtStCshnFldIsPosChk_Cal_sys/Subsystem2/Subsystem3 ==
  PosV : Inport
  Pos : Inport  Port=2
  CalibArray : Inport  Port=3
  Delta : Inport  Port=4
  Tolr : Inport  Port=5
  XXStIsPos_Get : FunctionCaller  FunctionPrototype=[IsPos,IsPosZone,IsPosAlready] = XXStIsPos_Get(PosV,Pos,CalibArray,Delta,Tolr)  InputArgumentSpecifications=boolean(true), uint16(1), uint16([1;1;1]), uint16(1), uint16(1)  OutputArgumentSpecifications=boolean(true), boolean(true), boolean(true)
  IsPos : Outport
  IsPosZone : Outport  Port=2
  IsPosAlready : Outport  Port=3
  wires:
  Pos/1 -> XXStIsPos_Get/2
  Delta/1 -> XXStIsPos_Get/4
  CalibArray/1 -> XXStIsPos_Get/3
  XXStIsPos_Get/2 -> IsPosZone/1
  XXStIsPos_Get/1 -> IsPos/1
  Tolr/1 -> XXStIsPos_Get/5
  XXStIsPos_Get/3 -> IsPosAlready/1
  PosV/1 -> XXStIsPos_Get/1

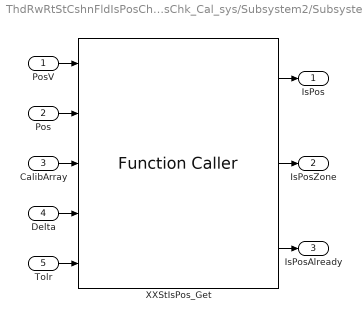
== system ThdRwRtStCshnFldIsPosChk/ThdRwRtStCshnFldIsPosChk_Cal_sys/Subsystem2/Subsystem4 ==
  PosV : Inport
  Pos : Inport  Port=2
  CalibArray : Inport  Port=3
  Delta : Inport  Port=4
  Tolr : Inport  Port=5
  XXStIsPos_Get : FunctionCaller  FunctionPrototype=[IsPos,IsPosZone,IsPosAlready] = XXStIsPos_Get(PosV,Pos,CalibArray,Delta,Tolr)  InputArgumentSpecifications=boolean(true), uint16(1), uint16([1;1;1]), uint16(1), uint16(1)  OutputArgumentSpecifications=boolean(true), boolean(true), boolean(true)
  IsPos : Outport
  IsPosZone : Outport  Port=2
  IsPosAlready : Outport  Port=3
  wires:
  PosV/1 -> XXStIsPos_Get/1
  XXStIsPos_Get/3 -> IsPosAlready/1
  Tolr/1 -> XXStIsPos_Get/5
  XXStIsPos_Get/1 -> IsPos/1
  XXStIsPos_Get/2 -> IsPosZone/1
  CalibArray/1 -> XXStIsPos_Get/3
  Delta/1 -> XXStIsPos_Get/4
  Pos/1 -> XXStIsPos_Get/2

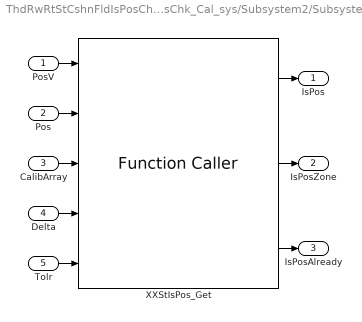
== system ThdRwRtStCshnFldIsPosChk/ThdRwRtStCshnFldIsPosChk_Cal_sys/Subsystem2/Subsystem5 ==
  PosV : Inport
  Pos : Inport  Port=2
  CalibArray : Inport  Port=3
  Delta : Inport  Port=4
  Tolr : Inport  Port=5
  XXStIsPos_Get : FunctionCaller  FunctionPrototype=[IsPos,IsPosZone,IsPosAlready] = XXStIsPos_Get(PosV,Pos,CalibArray,Delta,Tolr)  InputArgumentSpecifications=boolean(true), uint16(1), uint16([1;1;1]), uint16(1), uint16(1)  OutputArgumentSpecifications=boolean(true), boolean(true), boolean(true)
  IsPos : Outport
  IsPosZone : Outport  Port=2
  IsPosAlready : Outport  Port=3
  wires:
  PosV/1 -> XXStIsPos_Get/1
  XXStIsPos_Get/3 -> IsPosAlready/1
  Tolr/1 -> XXStIsPos_Get/5
  XXStIsPos_Get/1 -> IsPos/1
  XXStIsPos_Get/2 -> IsPosZone/1
  CalibArray/1 -> XXStIsPos_Get/3
  Delta/1 -> XXStIsPos_Get/4
  Pos/1 -> XXStIsPos_Get/2

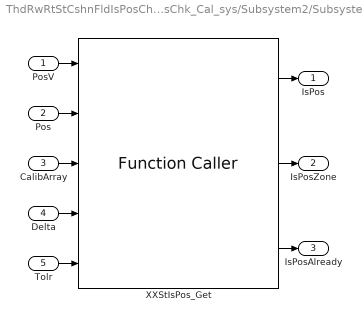
== system ThdRwRtStCshnFldIsPosChk/ThdRwRtStCshnFldIsPosChk_Cal_sys/Subsystem2/Subsystem6 ==
  PosV : Inport
  Pos : Inport  Port=2
  CalibArray : Inport  Port=3
  Delta : Inport  Port=4
  Tolr : Inport  Port=5
  XXStIsPos_Get : FunctionCaller  FunctionPrototype=[IsPos,IsPosZone,IsPosAlready] = XXStIsPos_Get(PosV,Pos,CalibArray,Delta,Tolr)  InputArgumentSpecifications=boolean(true), uint16(1), uint16([1;1;1]), uint16(1), uint16(1)  OutputArgumentSpecifications=boolean(true), boolean(true), boolean(true)
  IsPos : Outport
  IsPosZone : Outport  Port=2
  IsPosAlready : Outport  Port=3
  wires:
  Pos/1 -> XXStIsPos_Get/2
  Delta/1 -> XXStIsPos_Get/4
  CalibArray/1 -> XXStIsPos_Get/3
  XXStIsPos_Get/2 -> IsPosZone/1
  XXStIsPos_Get/1 -> IsPos/1
  Tolr/1 -> XXStIsPos_Get/5
  XXStIsPos_Get/3 -> IsPosAlready/1
  PosV/1 -> XXStIsPos_Get/1

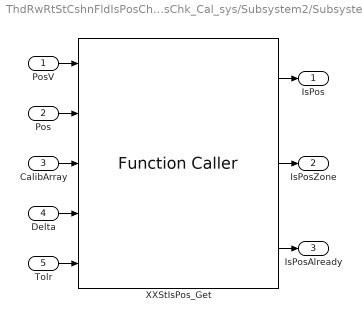
== system ThdRwRtStCshnFldIsPosChk/ThdRwRtStCshnFldIsPosChk_Cal_sys/Subsystem2/Subsystem7 ==
  PosV : Inport
  Pos : Inport  Port=2
  CalibArray : Inport  Port=3
  Delta : Inport  Port=4
  Tolr : Inport  Port=5
  XXStIsPos_Get : FunctionCaller  FunctionPrototype=[IsPos,IsPosZone,IsPosAlready] = XXStIsPos_Get(PosV,Pos,CalibArray,Delta,Tolr)  InputArgumentSpecifications=boolean(true), uint16(1), uint16([1;1;1]), uint16(1), uint16(1)  OutputArgumentSpecifications=boolean(true), boolean(true), boolean(true)
  IsPos : Outport
  IsPosZone : Outport  Port=2
  IsPosAlready : Outport  Port=3
  wires:
  PosV/1 -> XXStIsPos_Get/1
  XXStIsPos_Get/3 -> IsPosAlready/1
  Tolr/1 -> XXStIsPos_Get/5
  XXStIsPos_Get/1 -> IsPos/1
  XXStIsPos_Get/2 -> IsPosZone/1
  CalibArray/1 -> XXStIsPos_Get/3
  Delta/1 -> XXStIsPos_Get/4
  Pos/1 -> XXStIsPos_Get/2

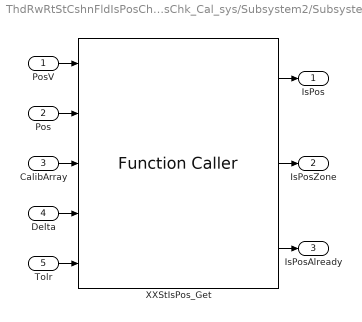
== system ThdRwRtStCshnFldIsPosChk/ThdRwRtStCshnFldIsPosChk_Cal_sys/Subsystem2/Subsystem8 ==
  PosV : Inport
  Pos : Inport  Port=2
  CalibArray : Inport  Port=3
  Delta : Inport  Port=4
  Tolr : Inport  Port=5
  XXStIsPos_Get : FunctionCaller  FunctionPrototype=[IsPos,IsPosZone,IsPosAlready] = XXStIsPos_Get(PosV,Pos,CalibArray,Delta,Tolr)  InputArgumentSpecifications=boolean(true), uint16(1), uint16([1;1;1]), uint16(1), uint16(1)  OutputArgumentSpecifications=boolean(true), boolean(true), boolean(true)
  IsPos : Outport
  IsPosZone : Outport  Port=2
  IsPosAlready : Outport  Port=3
  wires:
  PosV/1 -> XXStIsPos_Get/1
  XXStIsPos_Get/3 -> IsPosAlready/1
  Tolr/1 -> XXStIsPos_Get/5
  XXStIsPos_Get/1 -> IsPos/1
  XXStIsPos_Get/2 -> IsPosZone/1
  CalibArray/1 -> XXStIsPos_Get/3
  Delta/1 -> XXStIsPos_Get/4
  Pos/1 -> XXStIsPos_Get/2
